simulink model "controller_comb"  (R2020a)
settings: Solver=FixedStepAuto  StartTime=0.0  StopTime=50  FixedStep=0.001  RelTol=1e-3
values from neighbouring files (symbols this model uses):
  ss1 = ss(K1)    [lpv_config.m]
  ss2 = ss(K2)    [lpv_config.m]
  sysP = ss(P)    [lpv_config.m]
undefined symbols (not defined in the file or in its folder): options
libraries: simulink x7, cstblocks x1
settings Model: Creator=kekatos  LastModifiedBy=kekatos
settings DataIOCC: SignalLogging=off  DSMLogging=off  ReturnWorkspaceOutputs=off

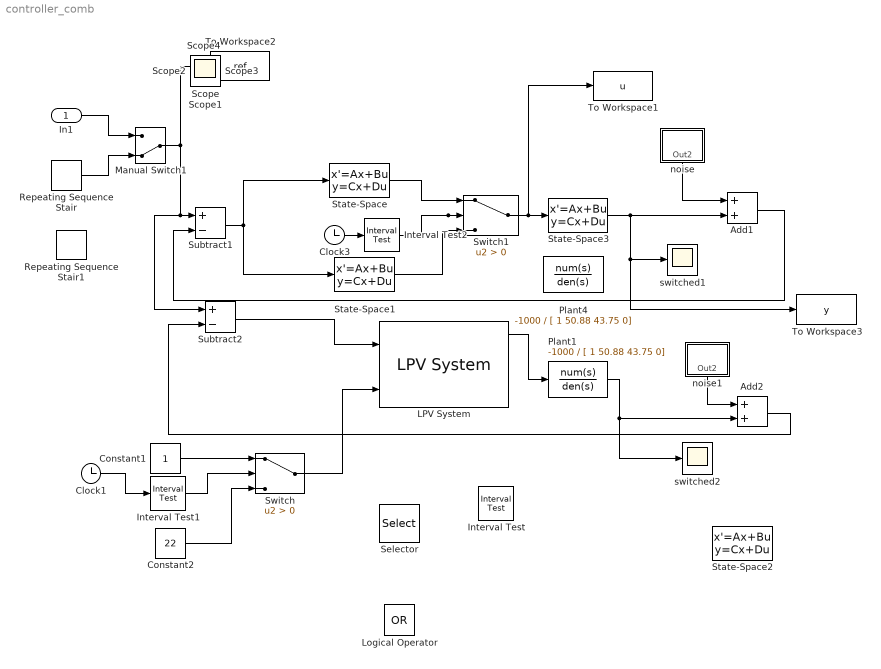
== system controller_comb ==
  In1 : Inport
  Add1 : Sum
  Add2 : Sum
  Clock1 : Clock
  Clock3 : Clock
  Constant1 : Constant
  Constant2 : Constant  Value=22
  Interval Test : simulink/Logic and Bit Operations/Interval Test  IntervalClosedRight=on  uplimit=0.5  IntervalClosedLeft=on  lowlimit=-0.5  OutDataTypeStr=boolean
  Interval Test1 : simulink/Logic and Bit Operations/Interval Test  IntervalClosedRight=on  uplimit=50  IntervalClosedLeft=on  lowlimit=25  OutDataTypeStr=boolean
  Interval Test2 : simulink/Logic and Bit Operations/Interval Test  IntervalClosedRight=on  uplimit=40  IntervalClosedLeft=on  lowlimit=18  OutDataTypeStr=boolean
  LPV System : cstblocks/Linear Parameter Varying/LPV System  sys=sys  x0=0  uOffset=0  yOffset=0  xOffset=0  opEquilOption=on  dxOffset=0  sysFixedOption=Use the first model in state-space array  sysFixed=[]  AFixed=false  BFixed=false  CFixed=false  DFixed=false  uDelayFixed=false  yDelayFixed=false  iDelayFixed=false  IMethod=Nearest  EMethod=Clip  IndexSearch=Binary search  IndexBegin=on  OutputX=on  OutputXdot=on  OutputLTI=on  OutputOP=on  DataType=double  SimMode=Interpreted execution  InitBufferSize=1024  FixedBuffer=off
      settings: SourceProductBaseCode=CT
  Logical Operator : Logic  Operator=OR  AllPortsSameDT=off  OutDataTypeStr=boolean
  Manual Switch1 : ManualSwitch  CurrentSetting=0
  Plant1 : TransferFcn  Numerator=-1000  Denominator=[ 1 50.88 43.75 0]
  Plant4 : TransferFcn  Numerator=-1000  Denominator=[ 1 50.88 43.75 0]
  Repeating Sequence Stair : simulink/Sources/Repeating Sequence Stair  OutValues=[1 0].'  tsamp=10  OutMin=[]  OutMax=[]  OutDataTypeStr=double  OutputDataTypeScalingMode=double  OutDataType=fixdt(0,8)  ConRadixGroup=Best Precision: Vector-wise  OutScaling=2^-12
  Repeating Sequence Stair1 : simulink/Sources/Repeating Sequence Stair  OutValues=[1;2]  tsamp=25  OutMin=[]  OutMax=[]  OutDataTypeStr=double  OutputDataTypeScalingMode=double  OutDataType=fixdt(0,8)  ConRadixGroup=Best Precision: Vector-wise  OutScaling=2^-12
  Selector : Selector  InputPortWidth=1  IndexOptions=Index vector (dialog)  Indices=[1]  OutputSizes=1
  State-Space : StateSpace  A=ss1.A  B=ss1.B  C=ss1.C  D=ss1.D  InitialCondition=0
  State-Space1 : StateSpace  A=ss2.A  B=ss2.B  C=ss2.C  D=ss2.D  InitialCondition=0
  State-Space2 : StateSpace  A=sysP.A  B=sysP.B  C=sysP.C  D=sysP.D  InitialCondition=0
  State-Space3 : StateSpace  A=sysP.A  B=sysP.B  C=sysP.C  D=sysP.D  InitialCondition=0
  Subtract1 : Sum  Inputs=+-
  Subtract2 : Sum  Inputs=+-
  Switch : Switch  Criteria=u2 > Threshold
  Switch1 : Switch  Criteria=u2 > Threshold
  To Workspace1 : ToWorkspace  VariableName=u  SaveFormat=Structure With Time  SampleTime=options.dt
  To Workspace2 : ToWorkspace  VariableName=ref  SaveFormat=Structure With Time  SampleTime=options.dt
  To Workspace3 : ToWorkspace  VariableName=y  SaveFormat=Structure With Time  SampleTime=options.dt
  noise : Subsystem
  noise1 : Subsystem
  switched1 : Scope
  switched2 : Scope
  Scope{,1..4} (5 alike) : Scope
  wires:
  Switch1/1 -> State-Space3/1, To Workspace1/1
  Interval Test2/1 -> Switch1/2
  Manual Switch1/1 -> Subtract2/1, Subtract1/1, To Workspace2/1
  Add1/1 -> Subtract1/2
  State-Space3/1 -> switched1/1, To Workspace3/1, Add1/2
  In1/1 -> Manual Switch1/1
  State-Space1/1 -> Switch1/3
  State-Space/1 -> Switch1/1
  Subtract1/1 -> State-Space1/1, State-Space/1
  Subtract2/1 -> LPV System/1
  LPV System/1 -> Plant1/1
  Plant1/1 -> switched2/1, Add2/2
  Add2/1 -> Subtract2/2
  Constant1/1 -> Switch/1
  Constant2/1 -> Switch/3
  Clock1/1 -> Interval Test1/1
  Interval Test1/1 -> Switch/2
  Switch/1 -> LPV System/2
  ? -> ?
  Clock3/1 -> Interval Test2/1
  noise/1(Out2) -> Add1/1
  noise1/1(Out2) -> Add2/1
  Repeating Sequence Stair/1 -> Manual Switch1/2

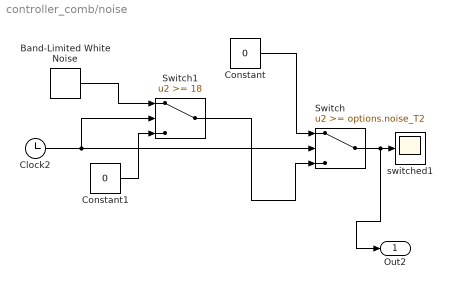
== system controller_comb/noise ==
  Band-Limited White Noise : simulink/Sources/Band-Limited White Noise  Cov=1e-5  Ts=options.dt  seed=[23341]
  Clock2 : Clock
  Constant : Constant  Value=0
  Constant1 : Constant  Value=0
  Switch : Switch  Threshold=options.noise_T2
  Switch1 : Switch  Threshold=18
  switched1 : Scope
  Out2 : Outport
  wires:
  Clock2/1 -> Switch1/2, Switch/2
  Constant/1 -> Switch/1
  Constant1/1 -> Switch1/3
  Band-Limited White Noise/1 -> Switch1/1
  Switch/1 -> Out2/1, switched1/1
  Switch1/1 -> Switch/3

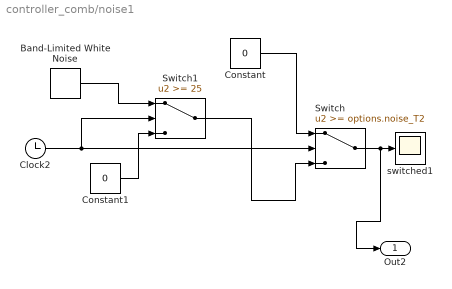
== system controller_comb/noise1 ==
  Band-Limited White Noise : simulink/Sources/Band-Limited White Noise  Cov=10^-6  Ts=options.dt  seed=[23341]
  Clock2 : Clock
  Constant : Constant  Value=0
  Constant1 : Constant  Value=0
  Switch : Switch  Threshold=options.noise_T2
  Switch1 : Switch  Threshold=25
  switched1 : Scope
  Out2 : Outport
  wires:
  Clock2/1 -> Switch1/2, Switch/2
  Constant/1 -> Switch/1
  Constant1/1 -> Switch1/3
  Band-Limited White Noise/1 -> Switch1/1
  Switch/1 -> Out2/1, switched1/1
  Switch1/1 -> Switch/3
